simulink model "sim"  (R2019b)
settings: Solver=ode23s  StartTime=0.0  StopTime=2.5  MaxStep=0.001  RelTol=1e-3
values from neighbouring files (symbols this model uses):
  A = [0 1 ... (first row only)    [semana 4 viernes.m]
  B = [1 0 ... (first row only)    [semana 4 viernes.m]
  C = [1 2]    [semana 4 viernes.m]
  D = [0 1]    [semana 4 viernes.m]
  GL = sysd.a    [semana 4 viernes.m]
  HL = sysd.b    [semana 4 viernes.m]
  Tm = 0.1    [semana 4 viernes.m]
  xini = [0.3; 0.1]    [semana 4 viernes.m]
settings Model: Creator=B13  LastModifiedBy=B13

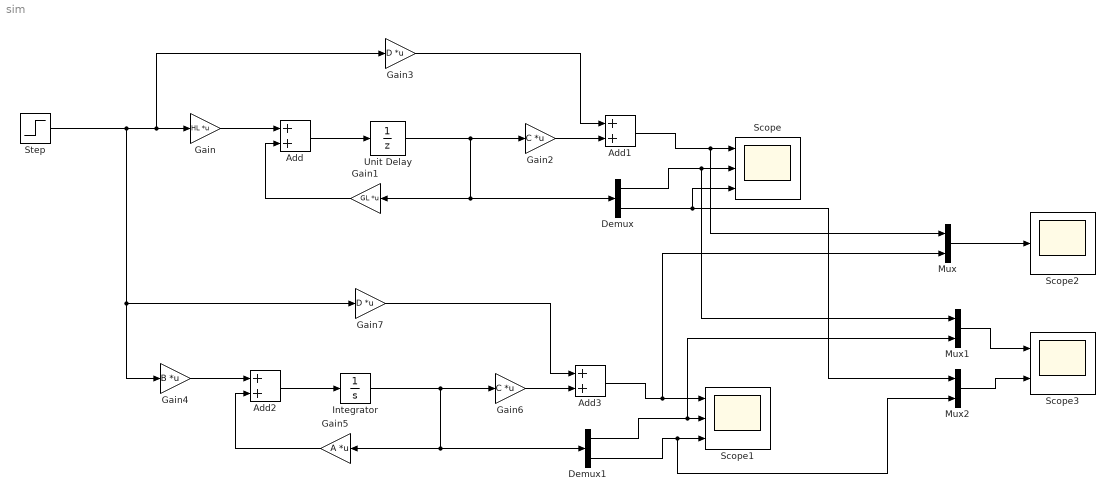
== system sim ==
  Add{,1..3} (4 alike) : Sum
  Demux : Demux  Outputs=2
  Demux1 : Demux  Outputs=2
  Gain : Gain  Gain=HL  Multiplication=Matrix(K*u)
  Gain1 : Gain  Gain=GL  Multiplication=Matrix(K*u)
  Gain2 : Gain  Gain=C  Multiplication=Matrix(K*u)
  Gain3 : Gain  Gain=D  Multiplication=Matrix(K*u)
  Gain4 : Gain  Gain=B  Multiplication=Matrix(K*u)
  Gain5 : Gain  Gain=A  Multiplication=Matrix(K*u)
  Gain6 : Gain  Gain=C  Multiplication=Matrix(K*u)
  Gain7 : Gain  Gain=D  Multiplication=Matrix(K*u)
  Integrator : Integrator  InitialCondition=xini
  Mux : Mux  Inputs=2
  Mux1 : Mux  Inputs=2
  Mux2 : Mux  Inputs=2
  Scope : Scope  NumInputPorts=3
  Scope1 : Scope  NumInputPorts=3
  Scope2 : Scope
  Scope3 : Scope  NumInputPorts=2
  Step : Step  After=[1;-2]  SampleTime=0
  Unit Delay : UnitDelay  InitialCondition=xini  SampleTime=Tm  HasFrameUpgradeWarning=on
  wires:
  Gain/1 -> Add/1
  Add/1 -> Unit Delay/1
  Gain1/1 -> Add/2
  Unit Delay/1 -> Gain2/1, Gain1/1, Demux/1
  Gain2/1 -> Add1/2
  Gain3/1 -> Add1/1
  Add1/1 -> Mux/1, Scope/1
  Demux/1 -> Mux1/1, Scope/2
  Demux/2 -> Mux2/1, Scope/3
  Gain6/1 -> Add3/2
  Gain5/1 -> Add2/2
  Gain7/1 -> Add3/1
  Integrator/1 -> Gain6/1, Gain5/1, Demux1/1
  Demux1/2 -> Mux2/2, Scope1/3
  Add2/1 -> Integrator/1
  Add3/1 -> Mux/2, Scope1/1
  Gain4/1 -> Add2/1
  Demux1/1 -> Mux1/2, Scope1/2
  Step/1 -> Gain4/1, Gain7/1, Gain3/1, Gain/1
  Mux/1 -> Scope2/1
  Mux1/1 -> Scope3/1
  Mux2/1 -> Scope3/2
